simulink model "EPT"  (R2019b)
settings: Solver=FixedStepDiscrete  StartTime=0.0  StopTime=5  FixedStep=0.005  RelTol=1e-3  EnableMultiTasking=on
PreLoadFcn:
  | try, model_open; catch, disp('Error occurred while executing model pre-load callback: model_open.m'); disp('Please assure that the MATLAB working directory is set to the model directory before opening.'); end
InitFcn:
  | try, model_open; catch, end
undefined symbols (not defined in the file or in its folder): Bridge, GCM, H, ln, raptor_get_param_eval, raptor_get_safe_string, raptor_xcp_function
libraries: Raptor_lib x2810, simulink x374, hdlsllib x19
(part 23 of 45)

== system EPT/Foreground_TimeBase_5ms/CHG//DCHG_PW_Control/EOC/Delay1/CycleTrigger ==
  In1 : Inport
  In2 : Inport  Port=2
  Add : Sum
  Add2 : Sum  Inputs=+-
  Constant2 : Constant  Value=0
  Constant3 : Constant
  Data Type Conversion1 : DataTypeConversion
  Data Type Conversion2 : DataTypeConversion
  Relational Operator1 : RelationalOperator  OutDataTypeStr=boolean  RndMeth=Simplest
  Saturation : Saturate  UpperLimit=inf  LowerLimit=2
  Switch : Switch  Threshold=1
  Unit Delay : UnitDelay  SampleTime=-1  HasFrameUpgradeWarning=on
  Trigger : Outport  VectorParamsAs1DForOutWhenUnconnected=off
  wires:
  Constant3/1 -> Add2/2
  In2/1 -> Saturation/1
  Add2/1 -> Data Type Conversion1/1
  Data Type Conversion2/1 -> Switch/2, Add/2
  Constant2/1 -> Switch/3
  Data Type Conversion1/1 -> Relational Operator1/2
  Relational Operator1/1 -> Trigger/1
  Switch/1 -> Unit Delay/1, Relational Operator1/1
  Unit Delay/1 -> Add/1
  In1/1 -> Data Type Conversion2/1
  Add/1 -> Switch/1
  Saturation/1 -> Add2/1

== system EPT/Foreground_TimeBase_5ms/CHG//DCHG_PW_Control/EOD/Delay1/CycleTrigger ==
  In1 : Inport
  In2 : Inport  Port=2
  Add : Sum
  Add2 : Sum  Inputs=+-
  Constant2 : Constant  Value=0
  Constant3 : Constant
  Data Type Conversion1 : DataTypeConversion
  Data Type Conversion2 : DataTypeConversion
  Relational Operator1 : RelationalOperator  OutDataTypeStr=boolean  RndMeth=Simplest
  Saturation : Saturate  UpperLimit=inf  LowerLimit=2
  Switch : Switch  Threshold=1
  Unit Delay : UnitDelay  SampleTime=-1  HasFrameUpgradeWarning=on
  Trigger : Outport  VectorParamsAs1DForOutWhenUnconnected=off
  wires:
  Constant3/1 -> Add2/2
  In2/1 -> Saturation/1
  Add2/1 -> Data Type Conversion1/1
  Data Type Conversion2/1 -> Switch/2, Add/2
  Constant2/1 -> Switch/3
  Data Type Conversion1/1 -> Relational Operator1/2
  Relational Operator1/1 -> Trigger/1
  Switch/1 -> Unit Delay/1, Relational Operator1/1
  Unit Delay/1 -> Add/1
  In1/1 -> Data Type Conversion2/1
  Add/1 -> Switch/1
  Saturation/1 -> Add2/1

== system EPT/Foreground_TimeBase_5ms/CHG//DCHG_PW_Control/Enhanced Coulomb Counting Algorithm/Coulomb Counting/20ms ==
  Ib : Inport
  Delta_DoD : Inport  Port=2
  Trigger : TriggerPort  VariantControl=Variant  PortDimensions=1
  Add2 : Sum
  Add3 : Sum
  Constant1 : Constant  Value=0
  Constant3 : Constant  Value=50
  Constant4 : Constant  Value=3600
  CountTrigger3 : Subsystem
  Delay1 : Delay  DelayLength=1  InitialCondition=0
  Divide1 : Product  Inputs=*/
  Divide3 : Product  Inputs=*/
  Switch1 : Switch  Criteria=u2 > Threshold
  Switch2 : Switch  Criteria=u2 > Threshold
  Delta DoD : Outport
  wires:
  Constant3/1 -> CountTrigger3/1(Counter), Divide3/2
  Delta_DoD/1 -> Add3/2
  Divide1/1 -> Add3/1
  Constant1/1 -> Switch2/3, Switch1/1
  Constant4/1 -> Divide1/2
  CountTrigger3/1(Tirgger) -> Switch1/2, Switch2/2
  Add2/1 -> Switch2/1, Switch1/3
  Switch1/1 -> Delay1/1
  Delay1/1 -> Add2/2
  Switch2/1 -> Divide1/1
  Divide3/1 -> Add2/1
  Ib/1 -> Divide3/1
  Add3/1 -> Delta DoD/1

== system EPT/Foreground_TimeBase_5ms/CHG//DCHG_PW_Control/Enhanced Coulomb Counting Algorithm/Coulomb Counting/CountTrigger ==
  Counter : Inport
  Constant1 : Constant  Value=0
  Constant3 : Constant
  CycleTrigger : Subsystem
  Switch : Switch  Threshold=1
  Unit Delay1 : UnitDelay  SampleTime=-1  HasFrameUpgradeWarning=on
  Unit Delay2 : UnitDelay  SampleTime=-1  HasFrameUpgradeWarning=on
  Tirgger : Outport  VectorParamsAs1DForOutWhenUnconnected=off
  wires:
  Switch/1 -> Unit Delay1/1
  Constant3/1 -> Switch/3
  Constant1/1 -> Switch/1
  Counter/1 -> CycleTrigger/2(In2)
  CycleTrigger/1(Trigger) -> Switch/2, Unit Delay2/1
  Unit Delay1/1 -> CycleTrigger/1(In1)
  Unit Delay2/1 -> Tirgger/1

== system EPT/Foreground_TimeBase_5ms/CHG//DCHG_PW_Control/Enhanced Coulomb Counting Algorithm Backup/Coulomb Counting1/20ms ==
  Ib : Inport
  Delta_DoD : Inport  Port=2
  Trigger : TriggerPort  VariantControl=Variant  PortDimensions=1
  Add2 : Sum
  Add3 : Sum
  Constant1 : Constant  Value=0
  Constant3 : Constant  Value=50
  Constant4 : Constant  Value=3600
  CountTrigger3 : Subsystem
  Delay1 : Delay  DelayLength=1  InitialCondition=0
  Divide1 : Product  Inputs=*/
  Divide3 : Product  Inputs=*/
  Switch1 : Switch  Criteria=u2 > Threshold
  Switch2 : Switch  Criteria=u2 > Threshold
  Delta DoD : Outport
  wires:
  Add3/1 -> Delta DoD/1
  Ib/1 -> Divide3/1
  Divide3/1 -> Add2/1
  Switch2/1 -> Divide1/1
  Delay1/1 -> Add2/2
  Switch1/1 -> Delay1/1
  Add2/1 -> Switch1/3, Switch2/1
  CountTrigger3/1(Tirgger) -> Switch2/2, Switch1/2
  Constant4/1 -> Divide1/2
  Constant1/1 -> Switch1/1, Switch2/3
  Divide1/1 -> Add3/1
  Delta_DoD/1 -> Add3/2
  Constant3/1 -> Divide3/2, CountTrigger3/1(Counter)

== system EPT/Foreground_TimeBase_5ms/CHG//DCHG_PW_Control/Enhanced Coulomb Counting Algorithm Backup/Coulomb Counting1/CountTrigger ==
  Counter : Inport
  Constant1 : Constant  Value=0
  Constant3 : Constant
  CycleTrigger : Subsystem
  Switch : Switch  Threshold=1
  Unit Delay1 : UnitDelay  SampleTime=-1  HasFrameUpgradeWarning=on
  Unit Delay2 : UnitDelay  SampleTime=-1  HasFrameUpgradeWarning=on
  Tirgger : Outport  VectorParamsAs1DForOutWhenUnconnected=off
  wires:
  Unit Delay2/1 -> Tirgger/1
  Unit Delay1/1 -> CycleTrigger/1(In1)
  CycleTrigger/1(Trigger) -> Unit Delay2/1, Switch/2
  Counter/1 -> CycleTrigger/2(In2)
  Constant1/1 -> Switch/1
  Constant3/1 -> Switch/3
  Switch/1 -> Unit Delay1/1

== system EPT/Foreground_TimeBase_5ms/CHG//DCHG_PW_Control/SWU Power Divider/PWCU/Latch1 ==
  Latch : Inport
  Reset : Inport  Port=2
  Switch1 : Switch  Criteria=u2 > Threshold
  Switch3 : Switch  Criteria=u2 > Threshold
  Unit Delay1 : UnitDelay  SampleTime=-1  HasFrameUpgradeWarning=on
  Output : Outport  VectorParamsAs1DForOutWhenUnconnected=off
  wires:
  Switch1/1 -> Switch3/3
  Latch/1 -> Switch1/2, Switch1/1
  Reset/1 -> Switch3/2
  Switch3/1 -> Unit Delay1/1, Output/1
  Unit Delay1/1 -> Switch1/3

== system EPT/Foreground_TimeBase_5ms/CHG//DCHG_PW_Control/SWU Power Divider/PWCU/Latch2 ==
  Latch : Inport
  Reset : Inport  Port=2
  Switch1 : Switch  Criteria=u2 > Threshold
  Switch3 : Switch  Criteria=u2 > Threshold
  Unit Delay1 : UnitDelay  SampleTime=-1  HasFrameUpgradeWarning=on
  Output : Outport  VectorParamsAs1DForOutWhenUnconnected=off
  wires:
  Switch1/1 -> Switch3/3
  Latch/1 -> Switch1/2, Switch1/1
  Reset/1 -> Switch3/2
  Switch3/1 -> Unit Delay1/1, Output/1
  Unit Delay1/1 -> Switch1/3

== system EPT/Foreground_TimeBase_5ms/E//W /BP-OBU_E//W/BP-OBU_E//W/BP-OBU_Fault_G4 ==
  "CMU_Work " : Inport
  Constant : Constant  Value=0
  Data Type Conversion{,1..3,5} (5 alike) : DataTypeConversion  OutDataTypeStr=uint8
  Fault CMU CAN ID : Subsystem
  Plus : Sum  Inputs=+++++
  Shift Arithmetic1 : ArithShift  BitShiftNumber=4  BitShiftDirection=Left
  Shift Arithmetic11 : ArithShift  BitShiftNumber=1  BitShiftDirection=Left
  Shift Arithmetic2 : ArithShift  BitShiftNumber=5  BitShiftDirection=Left
  Shift Arithmetic3 : ArithShift  BitShiftNumber=7  BitShiftDirection=Left
  Shift Arithmetic5 : ArithShift  BitShiftNumber=2  BitShiftDirection=Left
  raptor_data_def1 : Raptor_lib/Data Storage/raptor_data_def  dataName='BP_OBU_Fault_G4'  initValue=0  dataType=uint8  storage=Volatile (RAM)  calVisible=on  calType=Measurement  calDispType=Number  calEnum={'False', 'True'}  calGain=1.0  calOffset=0  calMin=-inf  calMax=inf  calFormat='-1'  calUnit=''  calHelp=''  calAccess=1  calFunction=raptor_xcp_function(gcb)  calDispHeaders=off  calColHeaders={'Col1' 'Col2' 'Col3'}  calRowHeaders={'Row1' 'Row2' 'Row3'}
      settings: SourceProductName=Raptor
  raptor_data_read1 : Raptor_lib/Data Storage/raptor_data_read  dataName='CAN_Fault_CMU2'  dataShape=Scalar  idxSource=Input  idxRow=1  idxCol=1
      settings: SourceProductName=Raptor
  raptor_data_read2 : Raptor_lib/Data Storage/raptor_data_read  dataName='CAN_Fault_CMU1'  dataShape=Scalar  idxSource=Input  idxRow=1  idxCol=1
      settings: SourceProductName=Raptor
  raptor_data_write : Raptor_lib/Data Storage/raptor_data_write  dataName='BP_OBU_Fault_G4'  dataShape=Scalar  idxSource=Input Port  idxRow=1  idxCol=1
      settings: SourceProductName=Raptor
  wires:
  Plus/1 -> raptor_data_write/1
  Data Type Conversion5/1 -> Shift Arithmetic3/1
  Shift Arithmetic3/1 -> Plus/5
  Constant/1 -> Data Type Conversion5/1
  Shift Arithmetic11/1 -> Plus/3
  Shift Arithmetic5/1 -> Plus/4
  Data Type Conversion1/1 -> Shift Arithmetic5/1
  Data Type Conversion/1 -> Shift Arithmetic11/1
  Fault CMU CAN ID/2(Fault_CMU2_CAN_ID) -> Data Type Conversion1/1
  "CMU_Work "/1 -> Fault CMU CAN ID/Enable
  Fault CMU CAN ID/1(Fault_CMU1_CAN_ID) -> Data Type Conversion/1
  Shift Arithmetic1/1 -> Plus/1
  raptor_data_read1/1 -> Data Type Conversion3/1
  raptor_data_read2/1 -> Data Type Conversion2/1
  Data Type Conversion2/1 -> Shift Arithmetic1/1
  Shift Arithmetic2/1 -> Plus/2
  Data Type Conversion3/1 -> Shift Arithmetic2/1

== system EPT/Foreground_TimeBase_5ms/E//W /BP-OBU_E//W/BP-OBU_E//W/BP-OBU_Warning//Fault_G1 ==
  Enable : EnablePort
  Add{,1..13} (14 alike) : Sum
  Data Type Conversion{,1..14,16} (16 alike) : DataTypeConversion  OutDataTypeStr=uint8
  Internal Res E/W : Subsystem
  SOC E/W : Subsystem
  Shift Arithmetic : ArithShift  BitShiftNumber=1  BitShiftDirection=Left
  Shift Arithmetic1 : ArithShift  BitShiftNumber=2  BitShiftDirection=Left
  Shift Arithmetic10 : ArithShift  BitShiftNumber=4  BitShiftDirection=Left
  Shift Arithmetic11 : ArithShift  BitShiftNumber=5  BitShiftDirection=Left
  Shift Arithmetic12 : ArithShift  BitShiftNumber=6  BitShiftDirection=Left
  Shift Arithmetic13 : ArithShift  BitShiftNumber=7  BitShiftDirection=Left
  Shift Arithmetic2 : ArithShift  BitShiftNumber=3  BitShiftDirection=Left
  Shift Arithmetic3 : ArithShift  BitShiftNumber=4  BitShiftDirection=Left
  Shift Arithmetic4 : ArithShift  BitShiftNumber=5  BitShiftDirection=Left
  Shift Arithmetic5 : ArithShift  BitShiftNumber=6  BitShiftDirection=Left
  Shift Arithmetic6 : ArithShift  BitShiftNumber=7  BitShiftDirection=Left
  Shift Arithmetic7 : ArithShift  BitShiftNumber=1  BitShiftDirection=Left
  Shift Arithmetic8 : ArithShift  BitShiftNumber=2  BitShiftDirection=Left
  Shift Arithmetic9 : ArithShift  BitShiftNumber=3  BitShiftDirection=Left
  Tbp E/W : Subsystem
  Vbp E/W : Subsystem
  raptor_data_def : Raptor_lib/Data Storage/raptor_data_def  dataName='BP_OBU_Warning_G1'  initValue=0  dataType=uint8  storage=Volatile (RAM)  calVisible=on  calType=Measurement  calDispType=Number  calEnum={'False', 'True'}  calGain=1.0  calOffset=0  calMin=-inf  calMax=inf  calFormat='-1'  calUnit=''  calHelp=''  calAccess=1  calFunction=raptor_xcp_function(gcb)  calDispHeaders=off  calColHeaders={'Col1' 'Col2' 'Col3'}  calRowHeaders={'Row1' 'Row2' 'Row3'}
      settings: SourceProductName=Raptor
  raptor_data_def1 : Raptor_lib/Data Storage/raptor_data_def  dataName='BP_OBU_Fault_G1'  initValue=0  dataType=uint8  storage=Volatile (RAM)  calVisible=on  calType=Measurement  calDispType=Number  calEnum={'False', 'True'}  calGain=1.0  calOffset=0  calMin=-inf  calMax=inf  calFormat='-1'  calUnit=''  calHelp=''  calAccess=1  calFunction=raptor_xcp_function(gcb)  calDispHeaders=off  calColHeaders={'Col1' 'Col2' 'Col3'}  calRowHeaders={'Row1' 'Row2' 'Row3'}
      settings: SourceProductName=Raptor
  raptor_data_write : Raptor_lib/Data Storage/raptor_data_write  dataName='BP_OBU_Warning_G1'  dataShape=Scalar  idxSource=Input Port  idxRow=1  idxCol=1
      settings: SourceProductName=Raptor
  raptor_data_write2 : Raptor_lib/Data Storage/raptor_data_write  dataName='BP_OBU_Fault_G1'  dataShape=Scalar  idxSource=Input Port  idxRow=1  idxCol=1
      settings: SourceProductName=Raptor
  wires:
  Vbp E/W/2(Warning_Vbp_High) -> Data Type Conversion1/1
  Internal Res E/W/1(Warning_Ichg_High) -> Data Type Conversion3/1
  Internal Res E/W/2(Warning_Idchg_High) -> Data Type Conversion4/1
  Tbp E/W/2(Warning_Tbp_Low_Temp) -> Data Type Conversion8/1
  Tbp E/W/1(Warning_Tbp_High_Temp) -> Data Type Conversion7/1
  SOC E/W/1(Warning_SOC_OutOfRange_High) -> Data Type Conversion11/1
  SOC E/W/2(Warning_SOC_OutOfRange_Low) -> Data Type Conversion12/1
  Vbp E/W/1(Warning_Vbp_Low) -> Data Type Conversion/1
  Shift Arithmetic/1 -> Add3/2
  Shift Arithmetic1/1 -> Add1/1
  Shift Arithmetic2/1 -> Add1/2
  Shift Arithmetic3/1 -> Add4/1
  Shift Arithmetic4/1 -> Add4/2
  Shift Arithmetic5/1 -> Add6/1
  Shift Arithmetic6/1 -> Add6/2
  Add3/1 -> Add11/1
  Add1/1 -> Add11/2
  Add4/1 -> Add8/1
  Add6/1 -> Add8/2
  Add11/1 -> Add12/1
  Add12/1 -> raptor_data_write/1
  Vbp E/W/4(Fault_Vbp_OV) -> Data Type Conversion2/1
  Vbp E/W/3(Fault_Vbp_UV) -> Data Type Conversion16/1
  Internal Res E/W/3(Fault_Ibp_OCC) -> Data Type Conversion5/1
  Internal Res E/W/4(Fault_Ibp_ODC) -> Data Type Conversion6/1
  Shift Arithmetic8/1 -> Add/1
  Shift Arithmetic9/1 -> Add/2
  Tbp E/W/3(Fault_Tbp_OT) -> Data Type Conversion9/1
  Tbp E/W/4(Fault_Tbp_UT) -> Data Type Conversion10/1
  Shift Arithmetic10/1 -> Add5/1
  Shift Arithmetic11/1 -> Add5/2
  SOC E/W/3(Fault_SOC_OutOfRange_High) -> Data Type Conversion13/1
  SOC E/W/4(Fault_SOC_OutOfRange_Low) -> Data Type Conversion14/1
  Shift Arithmetic12/1 -> Add7/1
  Shift Arithmetic13/1 -> Add7/2
  Add5/1 -> Add9/1
  Add7/1 -> Add9/2
  Add2/1 -> Add10/1
  Add/1 -> Add10/2
  Add10/1 -> Add13/1
  Add9/1 -> Add13/2
  Add13/1 -> raptor_data_write2/1
  Add8/1 -> Add12/2
  Data Type Conversion/1 -> Add3/1
  Data Type Conversion1/1 -> Shift Arithmetic/1
  Data Type Conversion16/1 -> Add2/1
  Data Type Conversion2/1 -> Shift Arithmetic7/1
  Data Type Conversion3/1 -> Shift Arithmetic1/1
  Data Type Conversion4/1 -> Shift Arithmetic2/1
  Data Type Conversion5/1 -> Shift Arithmetic8/1
  Data Type Conversion6/1 -> Shift Arithmetic9/1
  Data Type Conversion7/1 -> Shift Arithmetic3/1
  Data Type Conversion8/1 -> Shift Arithmetic4/1
  Data Type Conversion9/1 -> Shift Arithmetic10/1
  Data Type Conversion10/1 -> Shift Arithmetic11/1
  Data Type Conversion11/1 -> Shift Arithmetic5/1
  Data Type Conversion12/1 -> Shift Arithmetic6/1
  Data Type Conversion13/1 -> Shift Arithmetic12/1
  Data Type Conversion14/1 -> Shift Arithmetic13/1
  Shift Arithmetic7/1 -> Add2/2

== system EPT/Foreground_TimeBase_5ms/E//W /BP-OBU_E//W/BP-OBU_E//W/BP-OBU_Warning//Fault_G2 ==
  note: SOURCE:CAN3 Tx B2 &(BA-BB)
  Enable : EnablePort
  Add{,1..13} (14 alike) : Sum
  Data Type Conversion{1..16} (16 alike) : DataTypeConversion  OutDataTypeStr=uint8
  Shift Arithmetic : ArithShift  BitShiftNumber=1  BitShiftDirection=Left
  Shift Arithmetic1 : ArithShift  BitShiftNumber=2  BitShiftDirection=Left
  Shift Arithmetic10 : ArithShift  BitShiftNumber=6  BitShiftDirection=Left
  Shift Arithmetic11 : ArithShift  BitShiftNumber=5  BitShiftDirection=Left
  Shift Arithmetic12 : ArithShift  BitShiftNumber=3  BitShiftDirection=Left
  Shift Arithmetic13 : ArithShift  BitShiftNumber=7  BitShiftDirection=Left
  Shift Arithmetic2 : ArithShift  BitShiftNumber=3  BitShiftDirection=Left
  Shift Arithmetic3 : ArithShift  BitShiftNumber=4  BitShiftDirection=Left
  Shift Arithmetic4 : ArithShift  BitShiftNumber=5  BitShiftDirection=Left
  Shift Arithmetic5 : ArithShift  BitShiftNumber=6  BitShiftDirection=Left
  Shift Arithmetic6 : ArithShift  BitShiftNumber=7  BitShiftDirection=Left
  Shift Arithmetic7 : ArithShift  BitShiftNumber=1  BitShiftDirection=Left
  Shift Arithmetic8 : ArithShift  BitShiftNumber=4  BitShiftDirection=Left
  Shift Arithmetic9 : ArithShift  BitShiftNumber=2  BitShiftDirection=Left
  Tcell E/W : Subsystem
  Vcell E/W : Subsystem
  raptor_data_def : Raptor_lib/Data Storage/raptor_data_def  dataName='BP_OBU_Warning_G2'  initValue=0  dataType=uint8  storage=Volatile (RAM)  calVisible=on  calType=Measurement  calDispType=Number  calEnum={'False', 'True'}  calGain=1.0  calOffset=0  calMin=-inf  calMax=inf  calFormat='-1'  calUnit=''  calHelp=''  calAccess=1  calFunction=raptor_xcp_function(gcb)  calDispHeaders=off  calColHeaders={'Col1' 'Col2' 'Col3'}  calRowHeaders={'Row1' 'Row2' 'Row3'}
      settings: SourceProductName=Raptor
  raptor_data_def1 : Raptor_lib/Data Storage/raptor_data_def  dataName='BP_OBU_Fault_G2'  initValue=0  dataType=uint8  storage=Volatile (RAM)  calVisible=on  calType=Measurement  calDispType=Number  calEnum={'False', 'True'}  calGain=1.0  calOffset=0  calMin=-inf  calMax=inf  calFormat='-1'  calUnit=''  calHelp=''  calAccess=1  calFunction=raptor_xcp_function(gcb)  calDispHeaders=off  calColHeaders={'Col1' 'Col2' 'Col3'}  calRowHeaders={'Row1' 'Row2' 'Row3'}
      settings: SourceProductName=Raptor
  raptor_data_def2 : Raptor_lib/Data Storage/raptor_data_def  dataName='Fault_CMU'  initValue=0  dataType=boolean  storage=Volatile (RAM)  calVisible=on  calType=Measurement  calDispType=Number  calEnum={'False', 'True'}  calGain=1.0  calOffset=0  calMin=-inf  calMax=inf  calFormat='-1'  calUnit=''  calHelp=''  calAccess=1  calFunction=raptor_xcp_function(gcb)  calDispHeaders=off  calColHeaders={'Col1' 'Col2' 'Col3'}  calRowHeaders={'Row1' 'Row2' 'Row3'}
      settings: SourceProductName=Raptor
  raptor_data_read : Raptor_lib/Data Storage/raptor_data_read  dataName='Warning_EndOfCharge'  dataShape=Scalar  idxSource=Input  idxRow=1  idxCol=1
      settings: SourceProductName=Raptor
  raptor_data_read1 : Raptor_lib/Data Storage/raptor_data_read  dataName='Warning_EndOfDischarge'  dataShape=Scalar  idxSource=Input  idxRow=1  idxCol=1
      settings: SourceProductName=Raptor
  raptor_data_read2 : Raptor_lib/Data Storage/raptor_data_read  dataName='Fault_SOA_OutOfRange'  dataShape=Scalar  idxSource=Input  idxRow=1  idxCol=1
      settings: SourceProductName=Raptor
  raptor_data_read3 : Raptor_lib/Data Storage/raptor_data_read  dataName='Fault_CMU'  dataShape=Scalar  idxSource=Input  idxRow=1  idxCol=1
      settings: SourceProductName=Raptor
  raptor_data_write : Raptor_lib/Data Storage/raptor_data_write  dataName='BP_OBU_Warning_G2'  dataShape=Scalar  idxSource=Input Port  idxRow=1  idxCol=1
      settings: SourceProductName=Raptor
  raptor_data_write1 : Raptor_lib/Data Storage/raptor_data_write  dataName='BP_OBU_Fault_G2'  dataShape=Scalar  idxSource=Input Port  idxRow=1  idxCol=1
      settings: SourceProductName=Raptor
  wires:
  Vcell E/W/1(Warning_Vcell_High) -> Data Type Conversion14/1
  Vcell E/W/2(Warning_Vcell_Low) -> Data Type Conversion1/1
  Tcell E/W/1(Warning_Tcell_High) -> Data Type Conversion6/1
  Tcell E/W/2(Warning_Tcell_Low) -> Data Type Conversion7/1
  Tcell E/W/6(Fault_UnBalanced_Tcell) -> Data Type Conversion11/1
  Vcell E/W/6(Fault_UnBalanced_Vcell) -> Data Type Conversion5/1
  Shift Arithmetic/1 -> Add/2
  Shift Arithmetic1/1 -> Add1/1
  Shift Arithmetic2/1 -> Add1/2
  Tcell E/W/3(Warning_UnBalanced_Tcell) -> Data Type Conversion8/1
  Tcell E/W/4(Fault_Tcell_OT) -> Data Type Conversion9/1
  Vcell E/W/5(Warning_UnBalanced_Vcell) -> Data Type Conversion4/1
  Shift Arithmetic11/1 -> Add2/1
  Shift Arithmetic8/1 -> Add2/2
  Vcell E/W/4(Fault_Vcell_UV) -> Data Type Conversion3/1
  Vcell E/W/3(Fault_Vcell_OV) -> Data Type Conversion2/1
  Shift Arithmetic7/1 -> Add3/2
  Shift Arithmetic4/1 -> Add4/1
  Shift Arithmetic3/1 -> Add4/2
  Tcell E/W/5(Fault_Tcell_UT) -> Data Type Conversion10/1
  Shift Arithmetic12/1 -> Add5/2
  Shift Arithmetic9/1 -> Add5/1
  raptor_data_read1/1 -> Data Type Conversion13/1
  raptor_data_read/1 -> Data Type Conversion12/1
  Shift Arithmetic5/1 -> Add6/1
  Shift Arithmetic6/1 -> Add6/2
  Add/1 -> Add7/1
  Add1/1 -> Add7/2
  Add2/1 -> Add8/1
  Add6/1 -> Add8/2
  Add7/1 -> Add9/1
  Add8/1 -> Add9/2
  Add9/1 -> raptor_data_write/1
  Add3/1 -> Add10/1
  Add5/1 -> Add10/2
  Add4/1 -> Add11/1
  Add10/1 -> Add12/1
  Add11/1 -> Add12/2
  Add12/1 -> raptor_data_write1/1
  raptor_data_read2/1 -> Data Type Conversion15/1
  Shift Arithmetic10/1 -> Add13/1
  Add13/1 -> Add11/2
  Shift Arithmetic13/1 -> Add13/2
  raptor_data_read3/1 -> Data Type Conversion16/1
  Data Type Conversion14/1 -> Add/1
  Data Type Conversion1/1 -> Shift Arithmetic/1
  Data Type Conversion2/1 -> Add3/1
  Data Type Conversion3/1 -> Shift Arithmetic7/1
  Data Type Conversion4/1 -> Shift Arithmetic11/1
  Data Type Conversion5/1 -> Shift Arithmetic4/1
  Data Type Conversion6/1 -> Shift Arithmetic1/1
  Data Type Conversion7/1 -> Shift Arithmetic2/1
  Data Type Conversion8/1 -> Shift Arithmetic8/1
  Data Type Conversion9/1 -> Shift Arithmetic9/1
  Data Type Conversion10/1 -> Shift Arithmetic12/1
  Data Type Conversion11/1 -> Shift Arithmetic3/1
  Data Type Conversion12/1 -> Shift Arithmetic5/1
  Data Type Conversion13/1 -> Shift Arithmetic6/1
  Data Type Conversion15/1 -> Shift Arithmetic10/1
  Data Type Conversion16/1 -> Shift Arithmetic13/1

== system EPT/Foreground_TimeBase_5ms/E//W /BP-OBU_E//W/BP-OBU_E//W/BP-OBU_Warning//Fault_G3 ==
  BP-OBU_Fault_G3 : Subsystem
  BP-OBU_Warning_G3 : Subsystem
  Data Type Conversion{,1..12} (13 alike) : DataTypeConversion  OutDataTypeStr=uint8
  Plus : Sum  Inputs=++++++
  Plus1 : Sum  Inputs=++++++++
  Shift Arithmetic : ArithShift  BitShiftNumber=2  BitShiftDirection=Left
  Shift Arithmetic1 : ArithShift  BitShiftNumber=3  BitShiftDirection=Left
  Shift Arithmetic10 : ArithShift  BitShiftNumber=7  BitShiftDirection=Left
  Shift Arithmetic11 : ArithShift  BitShiftNumber=1  BitShiftDirection=Left
  Shift Arithmetic2 : ArithShift  BitShiftNumber=4  BitShiftDirection=Left
  Shift Arithmetic3 : ArithShift  BitShiftNumber=5  BitShiftDirection=Left
  Shift Arithmetic4 : ArithShift  BitShiftNumber=6  BitShiftDirection=Left
  Shift Arithmetic5 : ArithShift  BitShiftNumber=2  BitShiftDirection=Left
  Shift Arithmetic6 : ArithShift  BitShiftNumber=3  BitShiftDirection=Left
  Shift Arithmetic7 : ArithShift  BitShiftNumber=4  BitShiftDirection=Left
  Shift Arithmetic8 : ArithShift  BitShiftNumber=5  BitShiftDirection=Left
  Shift Arithmetic9 : ArithShift  BitShiftNumber=6  BitShiftDirection=Left
  raptor_data_def : Raptor_lib/Data Storage/raptor_data_def  dataName='BP_OBU_Warning_G3'  initValue=0  dataType=uint8  storage=Volatile (RAM)  calVisible=on  calType=Measurement  calDispType=Number  calEnum={'False', 'True'}  calGain=1.0  calOffset=0  calMin=-inf  calMax=inf  calFormat='-1'  calUnit=''  calHelp=''  calAccess=1  calFunction=raptor_xcp_function(gcb)  calDispHeaders=off  calColHeaders={'Col1' 'Col2' 'Col3'}  calRowHeaders={'Row1' 'Row2' 'Row3'}
      settings: SourceProductName=Raptor
  raptor_data_def1 : Raptor_lib/Data Storage/raptor_data_def  dataName='BP_OBU_Fault_G3'  initValue=0  dataType=uint8  storage=Volatile (RAM)  calVisible=on  calType=Measurement  calDispType=Number  calEnum={'False', 'True'}  calGain=1.0  calOffset=0  calMin=-inf  calMax=inf  calFormat='-1'  calUnit=''  calHelp=''  calAccess=1  calFunction=raptor_xcp_function(gcb)  calDispHeaders=off  calColHeaders={'Col1' 'Col2' 'Col3'}  calRowHeaders={'Row1' 'Row2' 'Row3'}
      settings: SourceProductName=Raptor
  raptor_data_write : Raptor_lib/Data Storage/raptor_data_write  dataName='BP_OBU_Warning_G3'  dataShape=Scalar  idxSource=Input Port  idxRow=1  idxCol=1
      settings: SourceProductName=Raptor
  raptor_data_write1 : Raptor_lib/Data Storage/raptor_data_write  dataName='BP_OBU_Fault_G3'  dataShape=Scalar  idxSource=Input Port  idxRow=1  idxCol=1
      settings: SourceProductName=Raptor
  wires:
  BP-OBU_Warning_G3/3(Warning_Cdrive_Open) -> Data Type Conversion1/1
  BP-OBU_Warning_G3/4(Warning_Cchg_Open) -> Data Type Conversion2/1
  BP-OBU_Warning_G3/5(Warning_Caux_Open) -> Data Type Conversion3/1
  BP-OBU_Warning_G3/6(Warning_Csp_Open) -> Data Type Conversion4/1
  BP-OBU_Warning_G3/2(Warning_CMU_Status) -> Data Type Conversion/1
  Data Type Conversion/1 -> Shift Arithmetic/1
  Data Type Conversion1/1 -> Shift Arithmetic1/1
  Data Type Conversion2/1 -> Shift Arithmetic2/1
  Data Type Conversion3/1 -> Shift Arithmetic3/1
  Data Type Conversion4/1 -> Shift Arithmetic4/1
  BP-OBU_Warning_G3/1(Warning_SOA_OutOfRange) -> Plus/1
  Shift Arithmetic/1 -> Plus/2
  Shift Arithmetic1/1 -> Plus/3
  Shift Arithmetic2/1 -> Plus/4
  Shift Arithmetic3/1 -> Plus/5
  Shift Arithmetic4/1 -> Plus/6
  Plus/1 -> raptor_data_write/1
  BP-OBU_Warning_G3/7(Fault_Cdrive_Open) -> Data Type Conversion5/1
  BP-OBU_Warning_G3/8(Fault_Cchg_Open) -> Data Type Conversion6/1
  BP-OBU_Warning_G3/9(Warning_Cdrive_Open3) -> Data Type Conversion7/1
  BP-OBU_Warning_G3/10(Fault_Csp_Open) -> Data Type Conversion8/1
  Data Type Conversion6/1 -> Shift Arithmetic11/1
  Data Type Conversion7/1 -> Shift Arithmetic5/1
  Data Type Conversion8/1 -> Shift Arithmetic6/1
  BP-OBU_Fault_G3/1(Fault_Impact_Open) -> Data Type Conversion9/1
  BP-OBU_Fault_G3/2(Fault_HV_Leakage) -> Data Type Conversion10/1
  BP-OBU_Fault_G3/3(Fault_Short_Circuit) -> Data Type Conversion11/1
  BP-OBU_Fault_G3/4(Fault_HV_Setup_Fault) -> Data Type Conversion12/1
  Shift Arithmetic11/1 -> Plus1/2
  Shift Arithmetic5/1 -> Plus1/3
  Shift Arithmetic6/1 -> Plus1/4
  Shift Arithmetic7/1 -> Plus1/5
  Data Type Conversion5/1 -> Plus1/1
  Shift Arithmetic8/1 -> Plus1/6
  Shift Arithmetic9/1 -> Plus1/7
  Shift Arithmetic10/1 -> Plus1/8
  Plus1/1 -> raptor_data_write1/1
  Data Type Conversion9/1 -> Shift Arithmetic7/1
  Data Type Conversion10/1 -> Shift Arithmetic8/1
  Data Type Conversion11/1 -> Shift Arithmetic9/1
  Data Type Conversion12/1 -> Shift Arithmetic10/1

== system EPT/Foreground_TimeBase_5ms/E//W /BP-OBU_E//W/BP-OBU_E//W/BP-OBU_Warning//Fault_G5 ==
  BP-OBU_Fault_G5 : Subsystem
  BP-OBU_Warning_G5 : Subsystem
  Delay37 : Subsystem
  Delay38 : Subsystem
  Delay39 : Subsystem
  Delay40 : Subsystem
  Delay41 : Subsystem
  Delay42 : Subsystem
  Delay43 : Subsystem
  Delay44 : Subsystem
  Latch42 : Subsystem
  Latch43 : Subsystem
  Latch44 : Subsystem
  Latch45 : Subsystem
  Latch46 : Subsystem
  Latch47 : Subsystem
  Latch48 : Subsystem
  Latch49 : Subsystem
  raptor_adjustment108 : Raptor_lib/Data Storage/raptor_adjustment  paramName='Fault_BCU_EW1_TimeCount'  nameSource=Parameter  initValue=20  dataType=double  storage=Calibration  calDispType=Number  calEnum={'False', 'True'}  calGain=1.0  calOffset=0.0  calMax=inf  calMin=-inf  calFormat='-1'  calUnit=''  calHelp=''  calAccess=1  calFunction=raptor_xcp_function(gcb)  calDispHeaders=off  calColHeaders={'Col1' 'Col2' 'Col3'}  calRowHeaders={'Row1' 'Row2' 'Row3'}
      settings: SourceProductName=Raptor
  raptor_adjustment109 : Raptor_lib/Data Storage/raptor_adjustment  paramName='BCU_EW1'  nameSource=Parameter  initValue=0  dataType=boolean  storage=Calibration  calDispType=Number  calEnum={'False', 'True'}  calGain=1.0  calOffset=0.0  calMax=inf  calMin=-inf  calFormat='-1'  calUnit=''  calHelp=''  calAccess=1  calFunction=raptor_xcp_function(gcb)  calDispHeaders=off  calColHeaders={'Col1' 'Col2' 'Col3'}  calRowHeaders={'Row1' 'Row2' 'Row3'}
      settings: SourceProductName=Raptor
  raptor_adjustment110 : Raptor_lib/Data Storage/raptor_adjustment  paramName='Fault_BCU_EW2_TimeCount'  nameSource=Parameter  initValue=20  dataType=double  storage=Calibration  calDispType=Number  calEnum={'False', 'True'}  calGain=1.0  calOffset=0.0  calMax=inf  calMin=-inf  calFormat='-1'  calUnit=''  calHelp=''  calAccess=1  calFunction=raptor_xcp_function(gcb)  calDispHeaders=off  calColHeaders={'Col1' 'Col2' 'Col3'}  calRowHeaders={'Row1' 'Row2' 'Row3'}
      settings: SourceProductName=Raptor
  raptor_adjustment111 : Raptor_lib/Data Storage/raptor_adjustment  paramName='BCU_EW2'  nameSource=Parameter  initValue=0  dataType=boolean  storage=Calibration  calDispType=Number  calEnum={'False', 'True'}  calGain=1.0  calOffset=0.0  calMax=inf  calMin=-inf  calFormat='-1'  calUnit=''  calHelp=''  calAccess=1  calFunction=raptor_xcp_function(gcb)  calDispHeaders=off  calColHeaders={'Col1' 'Col2' 'Col3'}  calRowHeaders={'Row1' 'Row2' 'Row3'}
      settings: SourceProductName=Raptor
  raptor_adjustment112 : Raptor_lib/Data Storage/raptor_adjustment  paramName='Fault_BCU_EW3_TimeCount'  nameSource=Parameter  initValue=20  dataType=double  storage=Calibration  calDispType=Number  calEnum={'False', 'True'}  calGain=1.0  calOffset=0.0  calMax=inf  calMin=-inf  calFormat='-1'  calUnit=''  calHelp=''  calAccess=1  calFunction=raptor_xcp_function(gcb)  calDispHeaders=off  calColHeaders={'Col1' 'Col2' 'Col3'}  calRowHeaders={'Row1' 'Row2' 'Row3'}
      settings: SourceProductName=Raptor
  raptor_adjustment113 : Raptor_lib/Data Storage/raptor_adjustment  paramName='BCU_EW3'  nameSource=Parameter  initValue=0  dataType=boolean  storage=Calibration  calDispType=Number  calEnum={'False', 'True'}  calGain=1.0  calOffset=0.0  calMax=inf  calMin=-inf  calFormat='-1'  calUnit=''  calHelp=''  calAccess=1  calFunction=raptor_xcp_function(gcb)  calDispHeaders=off  calColHeaders={'Col1' 'Col2' 'Col3'}  calRowHeaders={'Row1' 'Row2' 'Row3'}
      settings: SourceProductName=Raptor
  raptor_adjustment114 : Raptor_lib/Data Storage/raptor_adjustment  paramName='Fault_BCU_EW4_TimeCount'  nameSource=Parameter  initValue=20  dataType=double  storage=Calibration  calDispType=Number  calEnum={'False', 'True'}  calGain=1.0  calOffset=0.0  calMax=inf  calMin=-inf  calFormat='-1'  calUnit=''  calHelp=''  calAccess=1  calFunction=raptor_xcp_function(gcb)  calDispHeaders=off  calColHeaders={'Col1' 'Col2' 'Col3'}  calRowHeaders={'Row1' 'Row2' 'Row3'}
      settings: SourceProductName=Raptor
  raptor_adjustment115 : Raptor_lib/Data Storage/raptor_adjustment  paramName='BCU_EW4'  nameSource=Parameter  initValue=0  dataType=boolean  storage=Calibration  calDispType=Number  calEnum={'False', 'True'}  calGain=1.0  calOffset=0.0  calMax=inf  calMin=-inf  calFormat='-1'  calUnit=''  calHelp=''  calAccess=1  calFunction=raptor_xcp_function(gcb)  calDispHeaders=off  calColHeaders={'Col1' 'Col2' 'Col3'}  calRowHeaders={'Row1' 'Row2' 'Row3'}
      settings: SourceProductName=Raptor
  raptor_adjustment116 : Raptor_lib/Data Storage/raptor_adjustment  paramName='Fault_BCU_EW5_TimeCount'  nameSource=Parameter  initValue=20  dataType=double  storage=Calibration  calDispType=Number  calEnum={'False', 'True'}  calGain=1.0  calOffset=0.0  calMax=inf  calMin=-inf  calFormat='-1'  calUnit=''  calHelp=''  calAccess=1  calFunction=raptor_xcp_function(gcb)  calDispHeaders=off  calColHeaders={'Col1' 'Col2' 'Col3'}  calRowHeaders={'Row1' 'Row2' 'Row3'}
      settings: SourceProductName=Raptor
  raptor_adjustment117 : Raptor_lib/Data Storage/raptor_adjustment  paramName='BCU_EW5'  nameSource=Parameter  initValue=0  dataType=boolean  storage=Calibration  calDispType=Number  calEnum={'False', 'True'}  calGain=1.0  calOffset=0.0  calMax=inf  calMin=-inf  calFormat='-1'  calUnit=''  calHelp=''  calAccess=1  calFunction=raptor_xcp_function(gcb)  calDispHeaders=off  calColHeaders={'Col1' 'Col2' 'Col3'}  calRowHeaders={'Row1' 'Row2' 'Row3'}
      settings: SourceProductName=Raptor
  raptor_adjustment118 : Raptor_lib/Data Storage/raptor_adjustment  paramName='Fault_BCU_EW6_TimeCount'  nameSource=Parameter  initValue=20  dataType=double  storage=Calibration  calDispType=Number  calEnum={'False', 'True'}  calGain=1.0  calOffset=0.0  calMax=inf  calMin=-inf  calFormat='-1'  calUnit=''  calHelp=''  calAccess=1  calFunction=raptor_xcp_function(gcb)  calDispHeaders=off  calColHeaders={'Col1' 'Col2' 'Col3'}  calRowHeaders={'Row1' 'Row2' 'Row3'}
      settings: SourceProductName=Raptor
  raptor_adjustment119 : Raptor_lib/Data Storage/raptor_adjustment  paramName='BCU_EW6'  nameSource=Parameter  initValue=0  dataType=boolean  storage=Calibration  calDispType=Number  calEnum={'False', 'True'}  calGain=1.0  calOffset=0.0  calMax=inf  calMin=-inf  calFormat='-1'  calUnit=''  calHelp=''  calAccess=1  calFunction=raptor_xcp_function(gcb)  calDispHeaders=off  calColHeaders={'Col1' 'Col2' 'Col3'}  calRowHeaders={'Row1' 'Row2' 'Row3'}
      settings: SourceProductName=Raptor
  raptor_adjustment120 : Raptor_lib/Data Storage/raptor_adjustment  paramName='Fault_BCU_EW7_TimeCount'  nameSource=Parameter  initValue=20  dataType=double  storage=Calibration  calDispType=Number  calEnum={'False', 'True'}  calGain=1.0  calOffset=0.0  calMax=inf  calMin=-inf  calFormat='-1'  calUnit=''  calHelp=''  calAccess=1  calFunction=raptor_xcp_function(gcb)  calDispHeaders=off  calColHeaders={'Col1' 'Col2' 'Col3'}  calRowHeaders={'Row1' 'Row2' 'Row3'}
      settings: SourceProductName=Raptor
  raptor_adjustment121 : Raptor_lib/Data Storage/raptor_adjustment  paramName='BCU_EW7'  nameSource=Parameter  initValue=0  dataType=boolean  storage=Calibration  calDispType=Number  calEnum={'False', 'True'}  calGain=1.0  calOffset=0.0  calMax=inf  calMin=-inf  calFormat='-1'  calUnit=''  calHelp=''  calAccess=1  calFunction=raptor_xcp_function(gcb)  calDispHeaders=off  calColHeaders={'Col1' 'Col2' 'Col3'}  calRowHeaders={'Row1' 'Row2' 'Row3'}
      settings: SourceProductName=Raptor
  raptor_adjustment122 : Raptor_lib/Data Storage/raptor_adjustment  paramName='Fault_BCU_EW8_TimeCount'  nameSource=Parameter  initValue=20  dataType=double  storage=Calibration  calDispType=Number  calEnum={'False', 'True'}  calGain=1.0  calOffset=0.0  calMax=inf  calMin=-inf  calFormat='-1'  calUnit=''  calHelp=''  calAccess=1  calFunction=raptor_xcp_function(gcb)  calDispHeaders=off  calColHeaders={'Col1' 'Col2' 'Col3'}  calRowHeaders={'Row1' 'Row2' 'Row3'}
      settings: SourceProductName=Raptor
  raptor_adjustment123 : Raptor_lib/Data Storage/raptor_adjustment  paramName='BCU_EW8'  nameSource=Parameter  initValue=0  dataType=boolean  storage=Calibration  calDispType=Number  calEnum={'False', 'True'}  calGain=1.0  calOffset=0.0  calMax=inf  calMin=-inf  calFormat='-1'  calUnit=''  calHelp=''  calAccess=1  calFunction=raptor_xcp_function(gcb)  calDispHeaders=off  calColHeaders={'Col1' 'Col2' 'Col3'}  calRowHeaders={'Row1' 'Row2' 'Row3'}
      settings: SourceProductName=Raptor
  raptor_data_def1 : Raptor_lib/Data Storage/raptor_data_def  dataName='BP_OBU_Fault_G5'  initValue=0  dataType=uint8  storage=Volatile (RAM)  calVisible=on  calType=Measurement  calDispType=Number  calEnum={'False', 'True'}  calGain=1.0  calOffset=0  calMin=-inf  calMax=inf  calFormat='-1'  calUnit=''  calHelp=''  calAccess=1  calFunction=raptor_xcp_function(gcb)  calDispHeaders=off  calColHeaders={'Col1' 'Col2' 'Col3'}  calRowHeaders={'Row1' 'Row2' 'Row3'}
      settings: SourceProductName=Raptor
  raptor_data_read10 : Raptor_lib/Data Storage/raptor_data_read  dataName='MCU_InitFinishFlag'  dataShape=Scalar  idxSource=Input  idxRow=1  idxCol=1
      settings: SourceProductName=Raptor
  raptor_measurement40 : Raptor_lib/Data Storage/raptor_measurement  paramName='Fault_BCU_EW1'  nameSource=Parameter  calDispType=Number  calEnum={'False', 'True'}  calGain=1.0  calOffset=0.0  calMax=inf  calMin=-inf  calFormat='-1'  calUnit=''  calHelp=''  calAccess=1  calFunction=raptor_xcp_function(gcb)  calVisible=on
      settings: SourceProductName=Raptor
  raptor_measurement41 : Raptor_lib/Data Storage/raptor_measurement  paramName='Fault_BCU_EW2'  nameSource=Parameter  calDispType=Number  calEnum={'False', 'True'}  calGain=1.0  calOffset=0.0  calMax=inf  calMin=-inf  calFormat='-1'  calUnit=''  calHelp=''  calAccess=1  calFunction=raptor_xcp_function(gcb)  calVisible=on
      settings: SourceProductName=Raptor
  raptor_measurement42 : Raptor_lib/Data Storage/raptor_measurement  paramName='Fault_BCU_EW3'  nameSource=Parameter  calDispType=Number  calEnum={'False', 'True'}  calGain=1.0  calOffset=0.0  calMax=inf  calMin=-inf  calFormat='-1'  calUnit=''  calHelp=''  calAccess=1  calFunction=raptor_xcp_function(gcb)  calVisible=on
      settings: SourceProductName=Raptor
  raptor_measurement43 : Raptor_lib/Data Storage/raptor_measurement  paramName='Fault_BCU_EW4'  nameSource=Parameter  calDispType=Number  calEnum={'False', 'True'}  calGain=1.0  calOffset=0.0  calMax=inf  calMin=-inf  calFormat='-1'  calUnit=''  calHelp=''  calAccess=1  calFunction=raptor_xcp_function(gcb)  calVisible=on
      settings: SourceProductName=Raptor
  raptor_measurement44 : Raptor_lib/Data Storage/raptor_measurement  paramName='Fault_BCU_EW5'  nameSource=Parameter  calDispType=Number  calEnum={'False', 'True'}  calGain=1.0  calOffset=0.0  calMax=inf  calMin=-inf  calFormat='-1'  calUnit=''  calHelp=''  calAccess=1  calFunction=raptor_xcp_function(gcb)  calVisible=on
      settings: SourceProductName=Raptor
  raptor_measurement45 : Raptor_lib/Data Storage/raptor_measurement  paramName='Fault_BCU_EW6'  nameSource=Parameter  calDispType=Number  calEnum={'False', 'True'}  calGain=1.0  calOffset=0.0  calMax=inf  calMin=-inf  calFormat='-1'  calUnit=''  calHelp=''  calAccess=1  calFunction=raptor_xcp_function(gcb)  calVisible=on
      settings: SourceProductName=Raptor
  raptor_measurement46 : Raptor_lib/Data Storage/raptor_measurement  paramName='Fault_BCU_EW7'  nameSource=Parameter  calDispType=Number  calEnum={'False', 'True'}  calGain=1.0  calOffset=0.0  calMax=inf  calMin=-inf  calFormat='-1'  calUnit=''  calHelp=''  calAccess=1  calFunction=raptor_xcp_function(gcb)  calVisible=on
      settings: SourceProductName=Raptor
  raptor_measurement47 : Raptor_lib/Data Storage/raptor_measurement  paramName='Fault_BCU_EW8'  nameSource=Parameter  calDispType=Number  calEnum={'False', 'True'}  calGain=1.0  calOffset=0.0  calMax=inf  calMin=-inf  calFormat='-1'  calUnit=''  calHelp=''  calAccess=1  calFunction=raptor_xcp_function(gcb)  calVisible=on
      settings: SourceProductName=Raptor
  wires:
  Delay41/1(Output) -> Latch46/1(Latch)
  Delay42/1(Output) -> Latch47/1(Latch)
  raptor_adjustment117/1 -> Delay41/1(Condition)
  raptor_adjustment123/1 -> Delay44/1(Condition)
  raptor_adjustment122/1 -> Delay44/2(TimeCount)
  raptor_adjustment118/1 -> Delay42/2(TimeCount)
  raptor_adjustment116/1 -> Delay41/2(TimeCount)
  Latch43/1(Output) -> raptor_measurement41/1
  raptor_adjustment120/1 -> Delay43/2(TimeCount)
  Latch48/1(Output) -> raptor_measurement46/1
  raptor_adjustment121/1 -> Delay43/1(Condition)
  Delay43/1(Output) -> Latch48/1(Latch)
  Latch49/1(Output) -> raptor_measurement47/1
  Latch45/1(Output) -> raptor_measurement43/1
  raptor_adjustment110/1 -> Delay38/2(TimeCount)
  Delay38/1(Output) -> Latch43/1(Latch)
  Delay40/1(Output) -> Latch45/1(Latch)
  Latch47/1(Output) -> raptor_measurement45/1
  raptor_adjustment119/1 -> Delay42/1(Condition)
  raptor_adjustment114/1 -> Delay40/2(TimeCount)
  raptor_adjustment111/1 -> Delay38/1(Condition)
  Delay44/1(Output) -> Latch49/1(Latch)
  Delay39/1(Output) -> Latch44/1(Latch)
  Latch44/1(Output) -> raptor_measurement42/1
  raptor_adjustment113/1 -> Delay39/1(Condition)
  raptor_adjustment108/1 -> Delay37/2(TimeCount)
  Latch46/1(Output) -> raptor_measurement44/1
  raptor_adjustment112/1 -> Delay39/2(TimeCount)
  Delay37/1(Output) -> Latch42/1(Latch)
  raptor_adjustment115/1 -> Delay40/1(Condition)
  raptor_adjustment109/1 -> Delay37/1(Condition)
  Latch42/1(Output) -> raptor_measurement40/1
  raptor_data_read10/1 -> BP-OBU_Fault_G5/1("MCU Work "), BP-OBU_Warning_G5/1("MCU Work ")

== system EPT/Foreground_TimeBase_5ms/E//W /BP-OBU_E//W/Delay/CycleTrigger ==
  In1 : Inport
  In2 : Inport  Port=2
  Add : Sum
  Add2 : Sum  Inputs=+-
  Constant2 : Constant  Value=0
  Constant3 : Constant
  Data Type Conversion1 : DataTypeConversion
  Data Type Conversion2 : DataTypeConversion
  Relational Operator1 : RelationalOperator  OutDataTypeStr=boolean  RndMeth=Simplest
  Saturation : Saturate  UpperLimit=inf  LowerLimit=2
  Switch : Switch  Threshold=1
  Unit Delay : UnitDelay  SampleTime=-1  HasFrameUpgradeWarning=on
  Trigger : Outport  VectorParamsAs1DForOutWhenUnconnected=off
  wires:
  Saturation/1 -> Add2/1
  Add/1 -> Switch/1
  In1/1 -> Data Type Conversion2/1
  Unit Delay/1 -> Add/1
  Switch/1 -> Relational Operator1/1, Unit Delay/1
  Relational Operator1/1 -> Trigger/1
  Data Type Conversion1/1 -> Relational Operator1/2
  Constant2/1 -> Switch/3
  Data Type Conversion2/1 -> Add/2, Switch/2
  Add2/1 -> Data Type Conversion1/1
  In2/1 -> Saturation/1
  Constant3/1 -> Add2/2

== system EPT/Foreground_TimeBase_5ms/E//W /CAN_E//W/CAN_Abnormal/Warning ==
  " condition" : Inport
  Constant1 : Constant  Value=boolean('1')
  NOT1 : Logic  Operator=NOT  IconShape=distinctive  AllPortsSameDT=off  OutDataTypeStr=boolean
  Switch27 : Switch  Criteria=u2 > Threshold
  Warning : Outport  VectorParamsAs1DForOutWhenUnconnected=off
  wires:
  NOT1/1 -> Switch27/3
  Constant1/1 -> Switch27/1, NOT1/1
  " condition"/1 -> Switch27/2
  Switch27/1 -> Warning/1

== system EPT/Foreground_TimeBase_5ms/E//W /CAN_E//W/CAN_Abnormal/Warning1 ==
  " condition" : Inport
  Constant1 : Constant  Value=boolean('1')
  NOT1 : Logic  Operator=NOT  IconShape=distinctive  AllPortsSameDT=off  OutDataTypeStr=boolean
  Switch27 : Switch  Criteria=u2 > Threshold
  Warning : Outport  VectorParamsAs1DForOutWhenUnconnected=off
  wires:
  Switch27/1 -> Warning/1
  " condition"/1 -> Switch27/2
  Constant1/1 -> NOT1/1, Switch27/1
  NOT1/1 -> Switch27/3

== system EPT/Foreground_TimeBase_5ms/E//W /CAN_E//W/CAN_Abnormal/Warning10 ==
  " condition" : Inport
  Constant1 : Constant  Value=boolean('1')
  NOT1 : Logic  Operator=NOT  IconShape=distinctive  AllPortsSameDT=off  OutDataTypeStr=boolean
  Switch27 : Switch  Criteria=u2 > Threshold
  Warning : Outport  VectorParamsAs1DForOutWhenUnconnected=off
  wires:
  Switch27/1 -> Warning/1
  " condition"/1 -> Switch27/2
  Constant1/1 -> NOT1/1, Switch27/1
  NOT1/1 -> Switch27/3

== system EPT/Foreground_TimeBase_5ms/E//W /CAN_E//W/CAN_Abnormal/Warning11 ==
  " condition" : Inport
  Constant1 : Constant  Value=boolean('1')
  NOT1 : Logic  Operator=NOT  IconShape=distinctive  AllPortsSameDT=off  OutDataTypeStr=boolean
  Switch27 : Switch  Criteria=u2 > Threshold
  Warning : Outport  VectorParamsAs1DForOutWhenUnconnected=off
  wires:
  Switch27/1 -> Warning/1
  " condition"/1 -> Switch27/2
  Constant1/1 -> NOT1/1, Switch27/1
  NOT1/1 -> Switch27/3

== system EPT/Foreground_TimeBase_5ms/E//W /CAN_E//W/CAN_Abnormal/Warning12 ==
  " condition" : Inport
  Constant1 : Constant  Value=boolean('1')
  NOT1 : Logic  Operator=NOT  IconShape=distinctive  AllPortsSameDT=off  OutDataTypeStr=boolean
  Switch27 : Switch  Criteria=u2 > Threshold
  Warning : Outport  VectorParamsAs1DForOutWhenUnconnected=off
  wires:
  NOT1/1 -> Switch27/3
  Constant1/1 -> Switch27/1, NOT1/1
  " condition"/1 -> Switch27/2
  Switch27/1 -> Warning/1

== system EPT/Foreground_TimeBase_5ms/E//W /CAN_E//W/CAN_Abnormal/Warning2 ==
  " condition" : Inport
  Constant1 : Constant  Value=boolean('1')
  NOT1 : Logic  Operator=NOT  IconShape=distinctive  AllPortsSameDT=off  OutDataTypeStr=boolean
  Switch27 : Switch  Criteria=u2 > Threshold
  Warning : Outport  VectorParamsAs1DForOutWhenUnconnected=off
  wires:
  Switch27/1 -> Warning/1
  " condition"/1 -> Switch27/2
  Constant1/1 -> NOT1/1, Switch27/1
  NOT1/1 -> Switch27/3

== system EPT/Foreground_TimeBase_5ms/E//W /CAN_E//W/CAN_Abnormal/Warning3 ==
  " condition" : Inport
  Constant1 : Constant  Value=boolean('1')
  NOT1 : Logic  Operator=NOT  IconShape=distinctive  AllPortsSameDT=off  OutDataTypeStr=boolean
  Switch27 : Switch  Criteria=u2 > Threshold
  Warning : Outport  VectorParamsAs1DForOutWhenUnconnected=off
  wires:
  NOT1/1 -> Switch27/3
  Constant1/1 -> Switch27/1, NOT1/1
  " condition"/1 -> Switch27/2
  Switch27/1 -> Warning/1

== system EPT/Foreground_TimeBase_5ms/E//W /CAN_E//W/CAN_Abnormal/Warning4 ==
  " condition" : Inport
  Constant1 : Constant  Value=boolean('1')
  NOT1 : Logic  Operator=NOT  IconShape=distinctive  AllPortsSameDT=off  OutDataTypeStr=boolean
  Switch27 : Switch  Criteria=u2 > Threshold
  Warning : Outport  VectorParamsAs1DForOutWhenUnconnected=off
  wires:
  Switch27/1 -> Warning/1
  " condition"/1 -> Switch27/2
  Constant1/1 -> NOT1/1, Switch27/1
  NOT1/1 -> Switch27/3

== system EPT/Foreground_TimeBase_5ms/E//W /CAN_E//W/CAN_Abnormal/Warning5 ==
  " condition" : Inport
  Constant1 : Constant  Value=boolean('1')
  NOT1 : Logic  Operator=NOT  IconShape=distinctive  AllPortsSameDT=off  OutDataTypeStr=boolean
  Switch27 : Switch  Criteria=u2 > Threshold
  Warning : Outport  VectorParamsAs1DForOutWhenUnconnected=off
  wires:
  NOT1/1 -> Switch27/3
  Constant1/1 -> Switch27/1, NOT1/1
  " condition"/1 -> Switch27/2
  Switch27/1 -> Warning/1

== system EPT/Foreground_TimeBase_5ms/E//W /CAN_E//W/CAN_Abnormal/Warning6 ==
  " condition" : Inport
  Constant1 : Constant  Value=boolean('1')
  NOT1 : Logic  Operator=NOT  IconShape=distinctive  AllPortsSameDT=off  OutDataTypeStr=boolean
  Switch27 : Switch  Criteria=u2 > Threshold
  Warning : Outport  VectorParamsAs1DForOutWhenUnconnected=off
  wires:
  NOT1/1 -> Switch27/3
  Constant1/1 -> Switch27/1, NOT1/1
  " condition"/1 -> Switch27/2
  Switch27/1 -> Warning/1

== system EPT/Foreground_TimeBase_5ms/E//W /CAN_E//W/CAN_Abnormal/Warning7 ==
  " condition" : Inport
  Constant1 : Constant  Value=boolean('1')
  NOT1 : Logic  Operator=NOT  IconShape=distinctive  AllPortsSameDT=off  OutDataTypeStr=boolean
  Switch27 : Switch  Criteria=u2 > Threshold
  Warning : Outport  VectorParamsAs1DForOutWhenUnconnected=off
  wires:
  NOT1/1 -> Switch27/3
  Constant1/1 -> Switch27/1, NOT1/1
  " condition"/1 -> Switch27/2
  Switch27/1 -> Warning/1

== system EPT/Foreground_TimeBase_5ms/E//W /CAN_E//W/CAN_Abnormal/Warning8 ==
  " condition" : Inport
  Constant1 : Constant  Value=boolean('1')
  NOT1 : Logic  Operator=NOT  IconShape=distinctive  AllPortsSameDT=off  OutDataTypeStr=boolean
  Switch27 : Switch  Criteria=u2 > Threshold
  Warning : Outport  VectorParamsAs1DForOutWhenUnconnected=off
  wires:
  Switch27/1 -> Warning/1
  " condition"/1 -> Switch27/2
  Constant1/1 -> NOT1/1, Switch27/1
  NOT1/1 -> Switch27/3

== system EPT/Foreground_TimeBase_5ms/E//W /CAN_E//W/CAN_Abnormal/Warning9 ==
  " condition" : Inport
  Constant1 : Constant  Value=boolean('1')
  NOT1 : Logic  Operator=NOT  IconShape=distinctive  AllPortsSameDT=off  OutDataTypeStr=boolean
  Switch27 : Switch  Criteria=u2 > Threshold
  Warning : Outport  VectorParamsAs1DForOutWhenUnconnected=off
  wires:
  NOT1/1 -> Switch27/3
  Constant1/1 -> Switch27/1, NOT1/1
  " condition"/1 -> Switch27/2
  Switch27/1 -> Warning/1
